simulink model "Motor_position"  (R2020a)
settings: Solver=ode45  StartTime=0.0  StopTime=10.0  RelTol=1e-3
model workspace (MAT data in the model file):
  J = 3.2284e-06
  K = 0.0274
  L = 2.75e-06
  R = 4
  b = 3.5077e-06
settings Model: DataDictionary=prob4.sldd  Creator=HP  LastModifiedBy=Riyansh
settings DataIOCC: SaveOutput=off  SaveTime=off

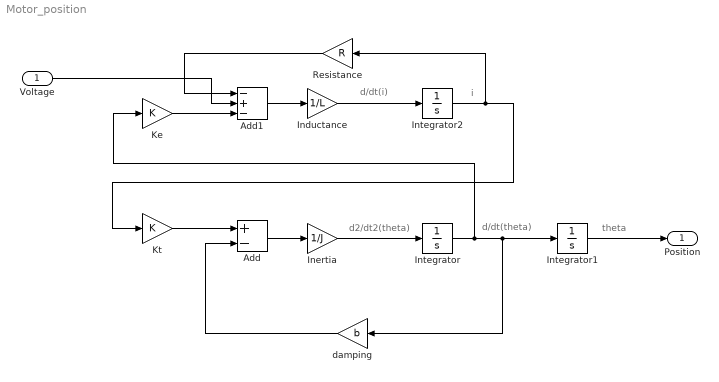
== system Motor_position ==
  note: i
  note: d/dt(i)
  note: d2/dt2(theta)
  note: d/dt(theta)
  note: theta
  Voltage : Inport  OutDataTypeStr=double  PortDimensions=1  SampleTime=0
  Add : Sum  Inputs=+-
  Add1 : Sum  Inputs=-+-
  Inductance : Gain  Gain=1/L
  Inertia : Gain  Gain=1/J
  Integrator : Integrator
  Integrator1 : Integrator
  Integrator2 : Integrator
  Ke : Gain  Gain=K
  Kt : Gain  Gain=K
  Resistance : Gain  Gain=R
  damping : Gain  Gain=b
  Position : Outport  OutDataTypeStr=double  PortDimensions=1  SampleTime=0
  wires:
  Inertia/1 -> Integrator/1
  Inductance/1 -> Integrator2/1
  Integrator2/1 -> Kt/1, Resistance/1
  Integrator/1 -> Integrator1/1, damping/1, Ke/1
  Integrator1/1 -> Position/1
  Voltage/1 -> Add1/2
  Add/1 -> Inertia/1
  damping/1 -> Add/2
  Kt/1 -> Add/1
  Resistance/1 -> Add1/1
  Ke/1 -> Add1/3
  Add1/1 -> Inductance/1
